simulink model "qc_posTest_fullstate"  (R2019b)
settings: Solver=VariableStepAuto  StartTime=0.0  StopTime=10.0  RelTol=1e-3
undefined symbols (not defined in the file or in its folder): param
settings Model: Creator=jorislegrand  LastModifiedBy=emiel

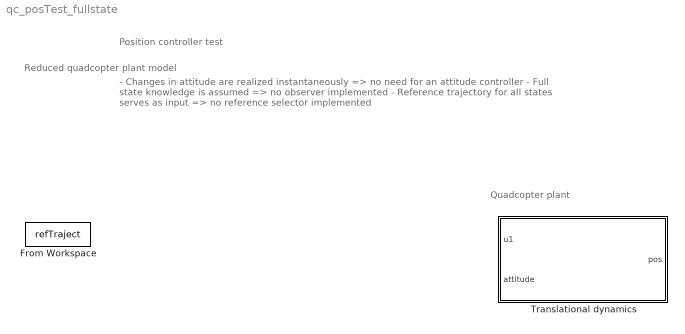
== system qc_posTest_fullstate ==
  note: Quadcopter plant
  note: - Changes in attitude are realized instantaneously => no need for an attitude controller
      | - Full state knowledge is assumed => no observer implemented
      | - Reference trajectory for all states serves as input => no reference selector implemented
  note: Position controller test
  note: Reduced quadcopter plant model
  From Workspace : FromWorkspace  VariableName=refTraject  SampleTime=0
  Translational dynamics : Subsystem

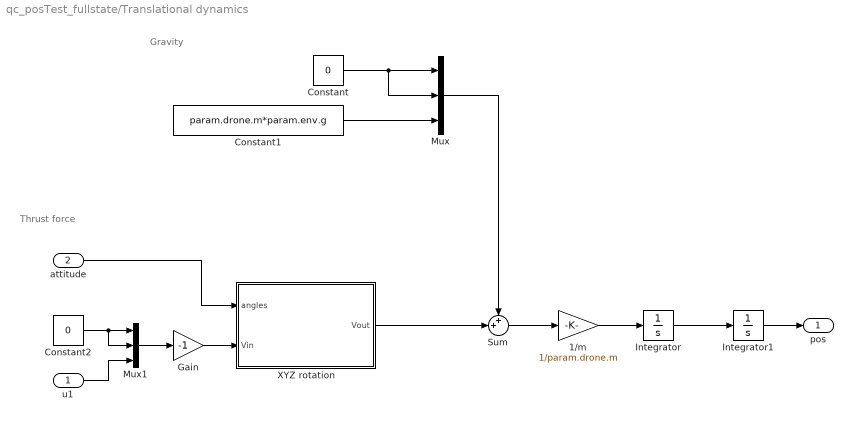
== system qc_posTest_fullstate/Translational dynamics ==
  note: Thrust force
  note: Gravity
  u1 : Inport
  attitude : Inport  Port=2
  1/m : Gain  Gain=1/param.drone.m
  Constant : Constant  Value=0
  Constant1 : Constant  Value=param.drone.m*param.env.g
  Constant2 : Constant  Value=0
  Gain : Gain  Gain=-1
  Integrator : Integrator  InitialCondition=param.x0.linvel
  Integrator1 : Integrator  InitialCondition=param.x0.pos
  Mux : Mux  Inputs=3
  Mux1 : Mux  Inputs=3
  Sum : Sum  Inputs=++|
  XYZ rotation : MATLAB Function  TreatAsAtomicUnit=on
  pos : Outport
  wires:
  attitude/1 -> XYZ rotation/1(angles)
  Constant/1 -> Mux/2, Mux/1
  Constant1/1 -> Mux/3
  XYZ rotation/1(Vout) -> Sum/2
  Mux/1 -> Sum/1
  Sum/1 -> 1/m/1
  Integrator/1 -> Integrator1/1
  Integrator1/1 -> pos/1
  1/m/1 -> Integrator/1
  Constant2/1 -> Mux1/2, Mux1/1
  u1/1 -> Mux1/3
  Mux1/1 -> Gain/1
  Gain/1 -> XYZ rotation/2(Vin)

== matlab function qc_posTest_fullstate/Translational dynamics/XYZ rotation ==
  data: angles input; Vout output; Vin input
function Vout = rotationXYZ(angles, Vin)
    R = eul2rotm(angles, 'XYZ');
    Vout = R*Vin;
